simulink model "free_floating_robot"  (R2017b)
settings: Solver=FixedStepAuto  StartTime=0.0  StopTime=10.0  FixedStep=0.01  RelTol=1e-3
settings Model: Creator=zhenya  LastModifiedBy=ernst
settings DataIOCC: ExternalInput=[t__, u__]  LoadExternalInput=on  SaveFormat=StructureWithTime

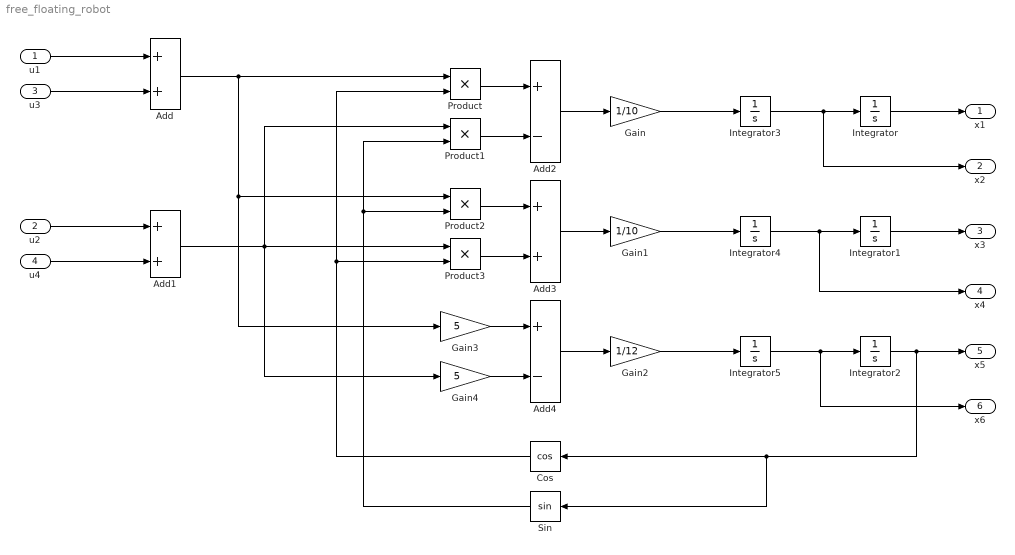
== system free_floating_robot ==
  u1 : Inport  Interpolate=off
  u2 : Inport  Port=2
  u3 : Inport  Port=3
  u4 : Inport  Port=4
  Add : Sum
  Add1 : Sum
  Add2 : Sum  Inputs=+-
  Add3 : Sum
  Add4 : Sum  Inputs=+-
  Cos : Trigonometry  Operator=cos
  Gain : Gain  Gain=1/10
  Gain1 : Gain  Gain=1/10
  Gain2 : Gain  Gain=1/12
  Gain3 : Gain  Gain=5
  Gain4 : Gain  Gain=5
  Integrator{,1..5} (6 alike) : Integrator
  Product{,1..3} (4 alike) : Product
  Sin : Trigonometry
  x1 : Outport
  x2 : Outport  Port=2
  x3 : Outport  Port=3
  x4 : Outport  Port=4
  x5 : Outport  Port=5
  x6 : Outport  Port=6
  wires:
  Add/1 -> Product/1, Gain3/1, Product2/1
  Integrator1/1 -> x3/1
  Gain4/1 -> Add4/2
  Gain1/1 -> Integrator4/1
  Gain/1 -> Integrator3/1
  Integrator2/1 -> Cos/1, Sin/1, x5/1
  u4/1 -> Add1/2
  u3/1 -> Add/2
  u2/1 -> Add1/1
  Add1/1 -> Gain4/1, Product3/1, Product1/1
  u1/1 -> Add/1
  Add3/1 -> Gain1/1
  Integrator/1 -> x1/1
  Sin/1 -> Product2/2, Product1/2
  Product2/1 -> Add3/1
  Add2/1 -> Gain/1
  Product/1 -> Add2/1
  Product3/1 -> Add3/2
  Add4/1 -> Gain2/1
  Cos/1 -> Product3/2, Product/2
  Gain2/1 -> Integrator5/1
  Product1/1 -> Add2/2
  Gain3/1 -> Add4/1
  Integrator3/1 -> x2/1, Integrator/1
  Integrator4/1 -> x4/1, Integrator1/1
  Integrator5/1 -> x6/1, Integrator2/1
